simulink model "PR6"  (R2014b)
settings: Solver=ode45  StartTime=0.0  StopTime=10.0  RelTol=1e-3
libraries: simulink_extras x2
settings Model: Creator=Najmol Anwar  LastModifiedBy=Najmol Anwar

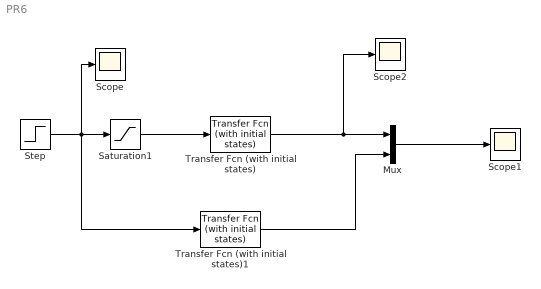
== system PR6 ==
  Mux : Mux  Inputs=2
  Saturation1 : Saturate  UpperLimit=5  LowerLimit=5
  Scope : Scope
  Scope1 : Scope
  Scope2 : Scope
      settings: SaveName=ScopeData2
  Step : Step  SampleTime=0
  Transfer Fcn (with initial states) : simulink_extras/Additional Linear/Transfer Fcn (with initial states)  N=[.2083]  D="[1  1.71]"  X0=.5
  Transfer Fcn (with initial states)1 : simulink_extras/Additional Linear/Transfer Fcn (with initial states)  N=[0.2083]  D="[1  1.71]"  X0=.5
  wires:
  Mux/1 -> Scope1/1
  Transfer Fcn (with initial states)/1 -> Scope2/1, Mux/1
  Transfer Fcn (with initial states)1/1 -> Mux/2
  Saturation1/1 -> Transfer Fcn (with initial states)/1
  Step/1 -> Transfer Fcn (with initial states)1/1, Saturation1/1, Scope/1
